simulink model "quad_model_control"  (R2025b)
settings: Solver=ode4  StartTime=0.0  StopTime=20  FixedStep=Ts/4  RelTol=1e-3
values from neighbouring files (symbols this model uses):
  axis_switch = [0 1 ... (first row only)    [quad_params.m]
  Cd = diag([0.10 0.10 0.15])    [quad_params.m]
  g = 9.81    [quad_params.m]
  Ivec = [Ixx; Iyy; Izz]    [quad_params.m]
  m = 1.20    (= 1.2)    [quad_params.m]
  MIX = [ kT     kT     kT     kT ... (first row only)    [quad_params.m]
  MIX_inv = inv(MIX)    [quad_params.m]
  ned_xy_kD = 1.92    [quad_params.m]
  ned_xy_kP = [1.44; 1.44]    [quad_params.m]
  ned_z_kD = 2.5    [quad_params.m]
  ned_z_kP = 2.7    [quad_params.m]
  om_dot_to_om = [0; 0; 0]    [quad_params.m]
  om_kP = [3;3;3]    [quad_params.m]
  p_ned_dot_to_p_ned = [0;0;0]    [quad_params.m]
  phi_dot_to_phi = [0;0;0]    [quad_params.m]
  pt1_w_cmd_to_w = zeros(4,1)    [quad_params.m]
  tau = 0.05    [quad_params.m]
  tau_kI = [0.125;0.125;0.324]    [quad_params.m]
  tau_kP = [0.10;0.10;0.216]    [quad_params.m]
  tau_sat_low = [-1.3;-1.3;-0.08]    [quad_params.m]
  tau_sat_up = [1.3;1.3;0.08]    [quad_params.m]
  Ts = 0.001    [quad_params.m]
  v_dot_to_v_b = [0;0;0]    [quad_params.m]
  w_max = 1200    [quad_params.m]
libraries: slpidlib x4
settings Model: Creator=chris  LastModifiedBy=chris
settings ModelReferenceCC: ModelReferenceMinAlgLoopOccurrences=on

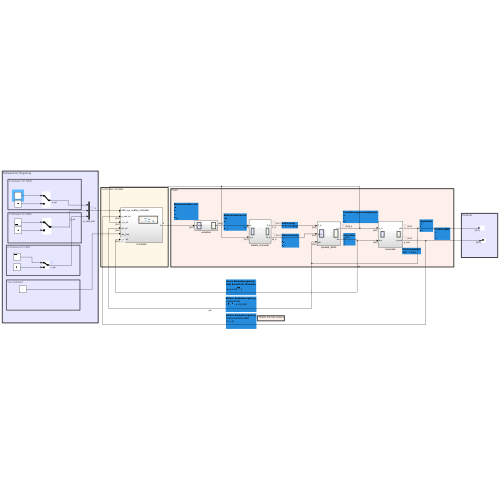
[thumbnail: Simulink's stored preview of the top-level diagram]
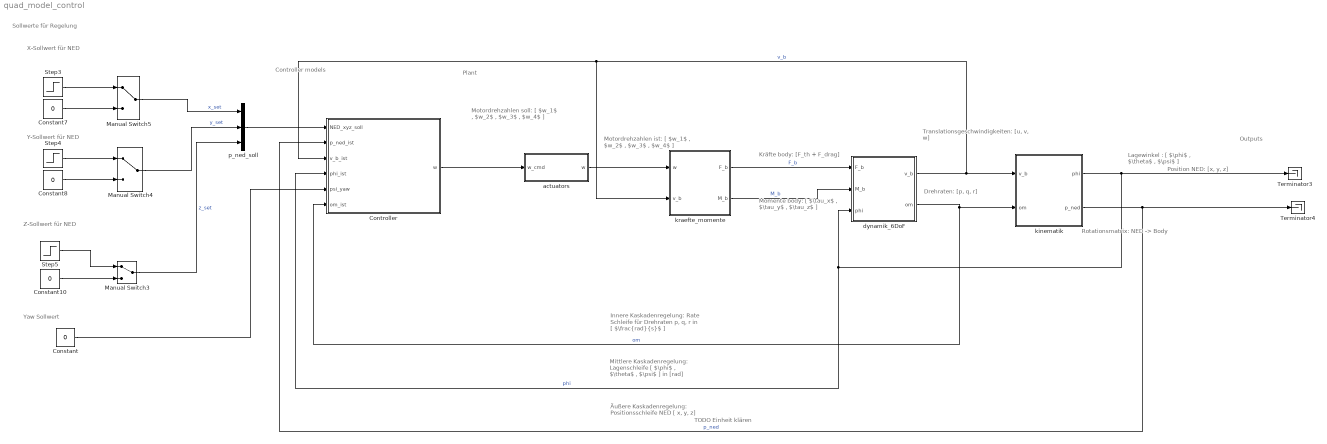
== system quad_model_control ==
  note: Controller models
  note: Plant
  note: Outputs
  note: Z-Sollwert für NED
  note: Sollwerte für Regelung
  note: Momente body:
      | [ $\tau_x$ ,
      | $\tau_y$ ,
      | $\tau_z$ ]
  note: Kräfte body:
      | [F_th + F_drag]
  note: Translationsgeschwindigkeiten:
      | [u,
      | v,
      | w]
  note: Drehraten:
      | [p,
      | q,
      | r]
  note: Lagewinkel :
      | [ $\phi$ ,
      | $\theta$ ,
      | $\psi$ ]
  note: Position NED:
      | [x,
      | y,
      | z]
  note: Rotationsmatrix:
      | NED -> Body
  note: Motordrehzahlen ist:
      | [ $w_1$ ,
      | $w_2$ ,
      | $w_3$ ,
      | $w_4$ ]
  note: Innere Kaskadenregelung:
      | Rate Schleife für Drehraten
      | p, q, r in [ $\frac{rad}{s}$ ]
  note: Mittlere Kaskadenregelung:
      | Lagenschleife
      | [ $\phi$ , $\theta$ , $\psi$ ] in [rad]
  note: Äußere Kaskadenregelung:
      | Positionsschleife NED
      | [ x, y, z]
  note: TODO Einheit klären
  note: X-Sollwert für NED
  note: Y-Sollwert für NED
  note: Motordrehzahlen soll:
      | [ $w_1$ ,
      | $w_2$ ,
      | $w_3$ ,
      | $w_4$ ]
  note: Yaw Sollwert
  Constant{,7..8,10} (4 alike) : Constant  Value=0
  Controller : Subsystem  Variant=on
  Manual Switch3 : ManualSwitch
  Manual Switch4 : ManualSwitch
  Manual Switch5 : ManualSwitch
  Step3 : Step  Time=2  After=2  SampleTime=0
  Step4 : Step  Time=2  After=2  SampleTime=0
  Step5 : Step  Time=2  After=-2  SampleTime=0
  Terminator3 : Terminator
  Terminator4 : Terminator
  actuators : Subsystem
  dynamik_6DoF : Subsystem
  kinematik : Subsystem
  kraefte_momente : Subsystem
  p_ned_soll : Mux  Inputs=3
  wires:
  dynamik_6DoF/2(om) -> Controller/6(om_ist), kinematik/2(om)  "om"
  kinematik/2(p_ned) -> Controller/2(p_ned_ist), Terminator4/1  "p_ned"
  kinematik/1(phi) -> dynamik_6DoF/3(phi), Controller/4(phi_ist), Terminator3/1  "phi"
  actuators/1(w) -> kraefte_momente/1(w)
  dynamik_6DoF/1(v_b) -> kinematik/1(v_b), Controller/3(v_b_ist), kraefte_momente/2(v_b)  "v_b"
  kraefte_momente/1(F_b) -> dynamik_6DoF/1(F_b)  "F_b"
  kraefte_momente/2(M_b) -> dynamik_6DoF/2(M_b)  "M_b"
  Constant8/1 -> Manual Switch4/2
  Step4/1 -> Manual Switch4/1
  Constant7/1 -> Manual Switch5/2
  Step3/1 -> Manual Switch5/1
  Manual Switch5/1 -> p_ned_soll/1  "x_set"
  Manual Switch4/1 -> p_ned_soll/2  "y_set"
  Step5/1 -> Manual Switch3/1
  Constant10/1 -> Manual Switch3/2
  Controller/1(w) -> actuators/1(w_cmd)
  p_ned_soll/1 -> Controller/1(NED_xyz_soll)
  Manual Switch3/1 -> p_ned_soll/3  "z_set"
  Constant/1 -> Controller/5(psi_yaw)

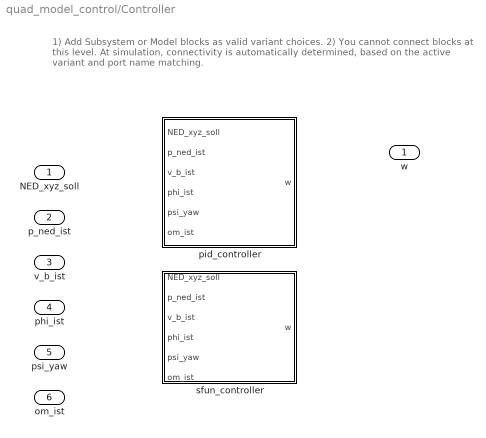
== system quad_model_control/Controller ==
  note: 1) Add Subsystem or Model blocks as valid variant choices.
      | 2) You cannot connect blocks at this level. At simulation, connectivity is automatically
      | determined, based on the active variant and port name matching.
  NED_xyz_soll : Inport
  p_ned_ist : Inport  Port=2
  v_b_ist : Inport  Port=3
  phi_ist : Inport  Port=4
  psi_yaw : Inport  Port=5
  om_ist : Inport  Port=6
  pid_controller : Subsystem  VariantControl=CTRL_IMPL ==1
  sfun_controller : Subsystem  VariantControl=CTRL_IMPL == 2
  w : Outport

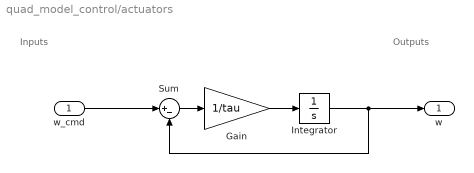
== system quad_model_control/actuators ==
  note: Inputs
  note: Outputs
  w_cmd : Inport  PortDimensions=[4 1]
  Gain : Gain  Gain=1/tau
  Integrator : Integrator  InitialCondition=pt1_w_cmd_to_w  LimitOutput=on  UpperSaturationLimit=w_max  LowerSaturationLimit=0  IgnoreLimit=on
  Sum : Sum  Inputs=|+-
  w : Outport  PortDimensions=[4 1]
  wires:
  Sum/1 -> Gain/1
  Gain/1 -> Integrator/1
  w_cmd/1 -> Sum/1
  Integrator/1 -> Sum/2, w/1

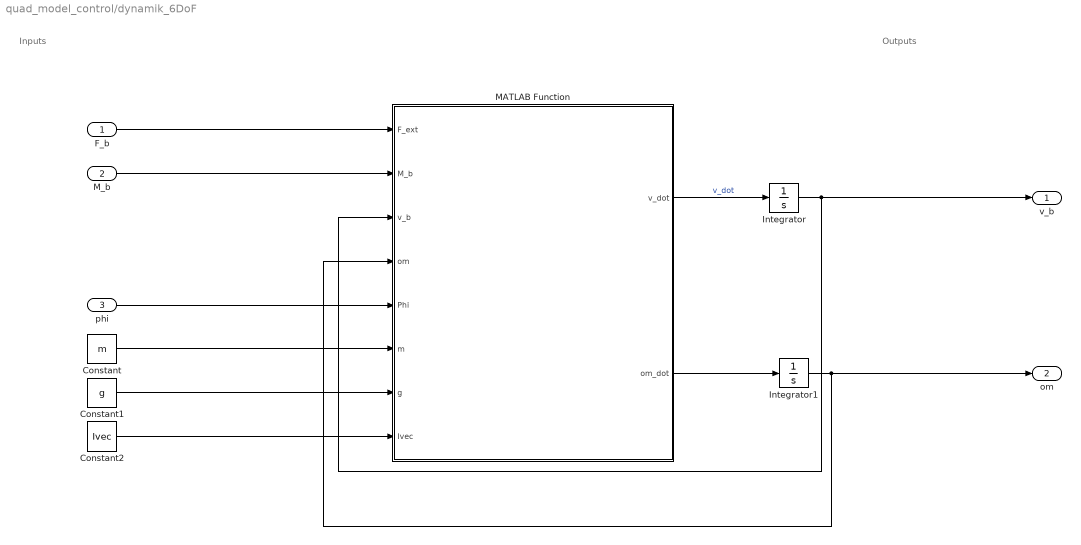
== system quad_model_control/dynamik_6DoF ==
  note: Inputs
  note: Outputs
  F_b : Inport  PortDimensions=[3 1]
  M_b : Inport  Port=2  PortDimensions=[3 1]
  phi : Inport  Port=3  PortDimensions=[3 1]
  Constant : Constant  Value=m
  Constant1 : Constant  Value=g
  Constant2 : Constant  Value=Ivec
  Integrator : Integrator  InitialCondition=v_dot_to_v_b
  Integrator1 : Integrator  InitialCondition=om_dot_to_om
  MATLAB Function : MATLAB Function  TreatAsAtomicUnit=on
  v_b : Outport  PortDimensions=[3 1]
  om : Outport  Port=2  PortDimensions=[3 1]
  wires:
  MATLAB Function/1(v_dot) -> Integrator/1  "v_dot"
  MATLAB Function/2(om_dot) -> Integrator1/1
  Constant1/1 -> MATLAB Function/7(g)
  F_b/1 -> MATLAB Function/1(F_ext)
  M_b/1 -> MATLAB Function/2(M_b)
  Constant/1 -> MATLAB Function/6(m)
  Integrator1/1 -> om/1, MATLAB Function/4(om)
  Constant2/1 -> MATLAB Function/8(Ivec)
  Integrator/1 -> v_b/1, MATLAB Function/3(v_b)
  phi/1 -> MATLAB Function/5(Phi)

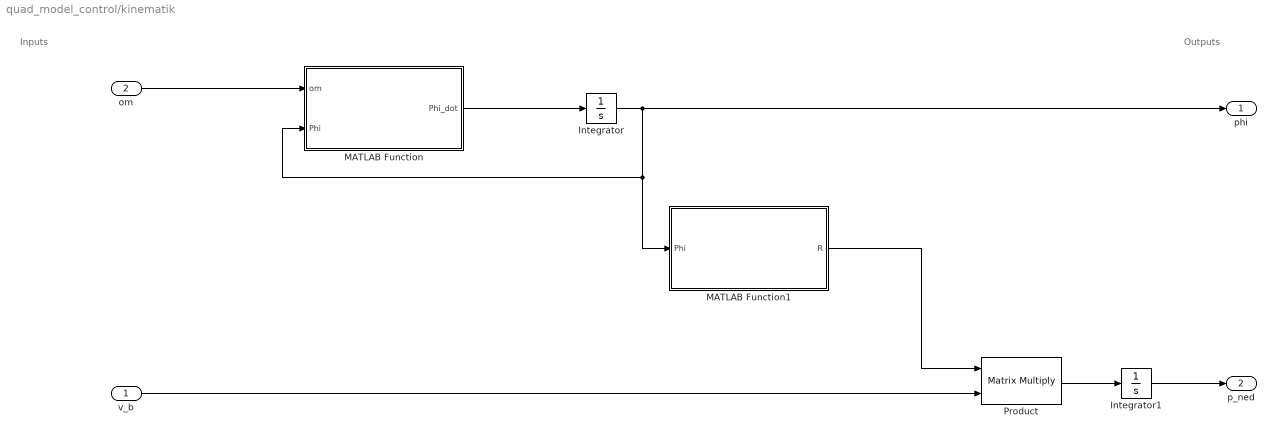
== system quad_model_control/kinematik ==
  note: Inputs
  note: Outputs
  v_b : Inport  PortDimensions=[3 1]
  om : Inport  Port=2  PortDimensions=[3 1]
  Integrator : Integrator  InitialCondition=phi_dot_to_phi
  Integrator1 : Integrator  InitialCondition=p_ned_dot_to_p_ned
  MATLAB Function : MATLAB Function  TreatAsAtomicUnit=on
  MATLAB Function1 : MATLAB Function  TreatAsAtomicUnit=on
  Product : Product  Multiplication=Matrix(*)
  phi : Outport  PortDimensions=[3 1]
  p_ned : Outport  Port=2
  wires:
  Integrator/1 -> phi/1, MATLAB Function1/1(Phi), MATLAB Function/2(Phi)
  Integrator1/1 -> p_ned/1
  v_b/1 -> Product/2
  MATLAB Function1/1(R) -> Product/1
  MATLAB Function/1(Phi_dot) -> Integrator/1
  om/1 -> MATLAB Function/1(om)
  Product/1 -> Integrator1/1

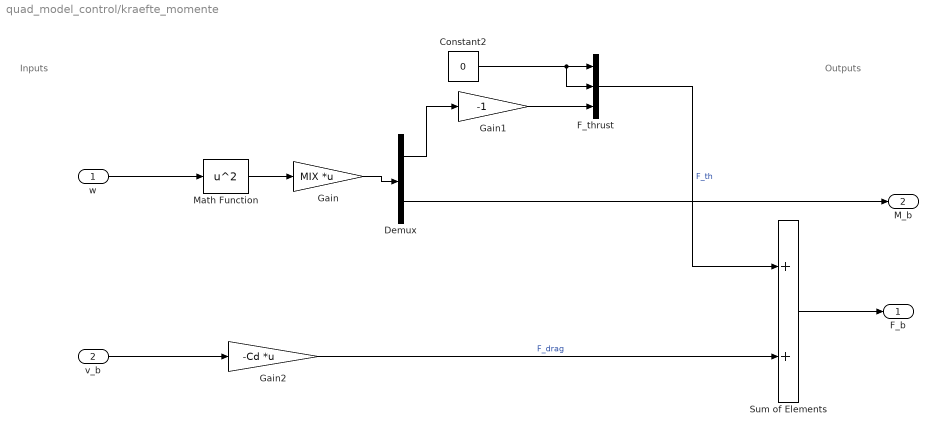
== system quad_model_control/kraefte_momente ==
  note: Inputs
  note: Outputs
  w : Inport  PortDimensions=[4 1]
  v_b : Inport  Port=2  PortDimensions=[3 1]
  Constant2 : Constant  Value=0
  Demux : Demux  Outputs=[1 3]
  F_thrust : Concatenate  NumInputs=3
  Gain : Gain  Gain=MIX  Multiplication=Matrix(K*u)
  Gain1 : Gain  Gain=-1
  Gain2 : Gain  Gain=-Cd  Multiplication=Matrix(K*u)
  Math Function : Math  Operator=square
  Sum of Elements : Sum
  F_b : Outport  PortDimensions=[3 1]
  M_b : Outport  Port=2  PortDimensions=[3 1]
  wires:
  v_b/1 -> Gain2/1
  Demux/2 -> M_b/1
  Constant2/1 -> F_thrust/2, F_thrust/1
  w/1 -> Math Function/1
  Gain2/1 -> Sum of Elements/2  "F_drag"
  Sum of Elements/1 -> F_b/1
  Math Function/1 -> Gain/1
  F_thrust/1 -> Sum of Elements/1  "F_th"
  Gain1/1 -> F_thrust/3
  Gain/1 -> Demux/1
  Demux/1 -> Gain1/1

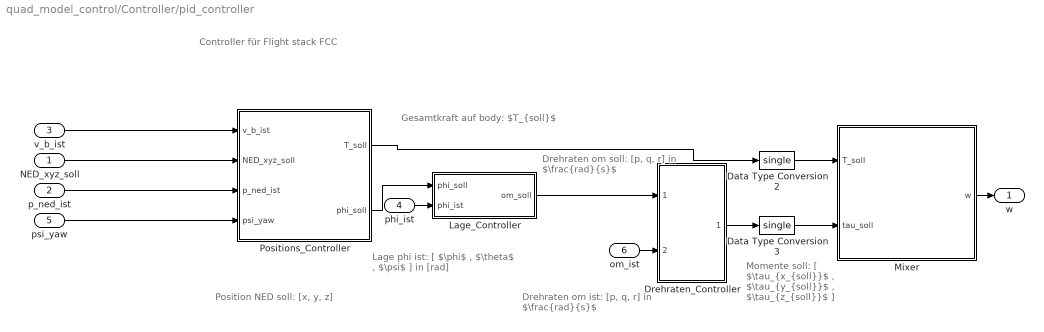
== system quad_model_control/Controller/pid_controller ==
  note: Controller für Flight stack FCC
  note: Drehraten om ist:
      | [p, q, r] in $\frac{rad}{s}$
  note: Lage phi ist:
      | [ $\phi$ , $\theta$ , $\psi$ ] in [rad]
  note: Momente soll:
      | [ $\tau_{x_{soll}}$ ,
      | $\tau_{y_{soll}}$ ,
      | $\tau_{z_{soll}}$ ]
  note: Gesamtkraft auf body:
      | $T_{soll}$
  note: Drehraten om soll:
      | [p, q, r] in $\frac{rad}{s}$
  note: Position NED soll:
      | [x, y, z]
  NED_xyz_soll : Inport
  p_ned_ist : Inport  Port=2
  v_b_ist : Inport  Port=3
  phi_ist : Inport  Port=4
  psi_yaw : Inport  Port=5
  om_ist : Inport  Port=6
  Data Type Conversion2 : DataTypeConversion  OutDataTypeStr=single  SaturateOnIntegerOverflow=off  RndMeth=Floor
  Data Type Conversion3 : DataTypeConversion  OutDataTypeStr=single  SaturateOnIntegerOverflow=off  RndMeth=Floor
  Drehraten_Controller : Subsystem
  Lage_Controller : Subsystem
  Mixer : Subsystem
  Positions_Controller : Subsystem
  w : Outport
  wires:
  psi_yaw/1 -> Positions_Controller/4(psi_yaw)
  Positions_Controller/2(phi_soll) -> Lage_Controller/1(phi_soll)
  Data Type Conversion2/1 -> Mixer/1(T_soll)
  Lage_Controller/1(om_soll) -> Drehraten_Controller/1(om_soll)
  Positions_Controller/1(T_soll) -> Data Type Conversion2/1
  Data Type Conversion3/1 -> Mixer/2(tau_soll)
  Mixer/1(w) -> w/1
  Drehraten_Controller/1(tau_soll) -> Data Type Conversion3/1
  phi_ist/1 -> Lage_Controller/2(phi_ist)
  v_b_ist/1 -> Positions_Controller/1(v_b_ist)
  p_ned_ist/1 -> Positions_Controller/3(p_ned_ist)
  om_ist/1 -> Drehraten_Controller/2(om_ist)
  NED_xyz_soll/1 -> Positions_Controller/2(NED_xyz_soll)

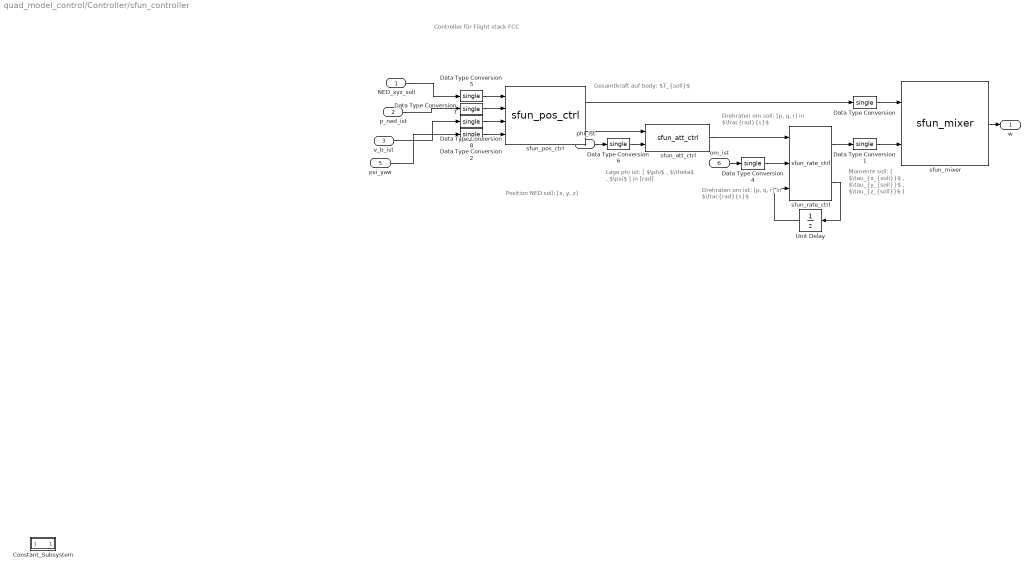
== system quad_model_control/Controller/sfun_controller ==
  note: Controller für Flight stack FCC
  note: Gesamtkraft auf body:
      | $T_{soll}$
  note: Drehraten om soll:
      | [p, q, r] in $\frac{rad}{s}$
  note: Drehraten om ist:
      | [p, q, r] in $\frac{rad}{s}$
  note: Lage phi ist:
      | [ $\phi$ , $\theta$ , $\psi$ ] in [rad]
  note: Position NED soll:
      | [x, y, z]
  note: Momente soll:
      | [ $\tau_{x_{soll}}$ ,
      | $\tau_{y_{soll}}$ ,
      | $\tau_{z_{soll}}$ ]
  NED_xyz_soll : Inport
  p_ned_ist : Inport  Port=2
  v_b_ist : Inport  Port=3
  phi_ist : Inport  Port=4
  psi_yaw : Inport  Port=5
  om_ist : Inport  Port=6
  Constant_Subsystem : Subsystem
  Data Type Conversion{,1..2,4..8} (8 alike) : DataTypeConversion  OutDataTypeStr=single  SaturateOnIntegerOverflow=off  RndMeth=Floor
  Unit Delay : UnitDelay  SampleTime=-1  HasFrameUpgradeWarning=on
  sfun_att_ctrl : S-Function  FunctionName=sfun_att_ctrl  SFunctionDeploymentMode=off  EnableBusSupport=off  mask(Legacy Function){SFunctionSpec=void att_ctrl_lct(single u1[3], single u2[3], single y1[3]), ShowSpec=on}
      mask prompts: ShowSpec "Display function specification"
      mask help:
      | This block allows you to call the legacy functions specified by the following Legacy Code Tool definition:
      | def.SFunctionName = 'sfun_att_ctrl';
      | def.OutputFcnSpec = 'void att_ctrl_lct(single u1[3], single u2[3], single y1[3])';
      | def.HeaderFiles = {'flight_ctrl_lct.h'};
      | def.SourceFiles = {'flight_ctrl.c', 'flight_ctrl_lct.c'};
      mask Help: <p>This block was generated automatically by the Legacy Code Tool. For detailed help on this tool, call<a href="matlab:legacy_code('help')"> legacy_code('help')</a>.</p>
      mask Callback ShowSpec:
      | if strcmp(get_param(gcbh, 'ShowSpec'), 'on')
      |   set_param(gcbh, 'MaskDisplay', sprintf('fprintf(''%s'');', get_param(gcbh, 'SFunctionSpec')));
      | else
      |   set_param(gcbh, 'MaskDisplay', sprintf('fprintf(''%s'');', get_param(gcbh, 'FunctionName')));
      | end
      mask Display: fprintf('void att_ctrl_lct(single u1[3], single u2[3], single y1[3])');
  sfun_mixer : S-Function  FunctionName=sfun_mixer  SFunctionDeploymentMode=off  EnableBusSupport=off  mask(Legacy Function){SFunctionSpec=void mixer_lct(single u1, single u2[3], single y1[4]), ShowSpec=on}
      mask prompts: ShowSpec "Display function specification"
      mask help:
      | This block allows you to call the legacy functions specified by the following Legacy Code Tool definition:
      | def.SFunctionName = 'sfun_mixer';
      | def.OutputFcnSpec = 'void mixer_lct(single u1, single u2[3], single y1[4])';
      | def.HeaderFiles = {'flight_ctrl_lct.h'};
      | def.SourceFiles = {'flight_ctrl.c', 'flight_ctrl_lct.c'};
      mask Help: <p>This block was generated automatically by the Legacy Code Tool. For detailed help on this tool, call<a href="matlab:legacy_code('help')"> legacy_code('help')</a>.</p>
      mask Callback ShowSpec:
      | if strcmp(get_param(gcbh, 'ShowSpec'), 'on')
      |   set_param(gcbh, 'MaskDisplay', sprintf('fprintf(''%s'');', get_param(gcbh, 'SFunctionSpec')));
      | else
      |   set_param(gcbh, 'MaskDisplay', sprintf('fprintf(''%s'');', get_param(gcbh, 'FunctionName')));
      | end
      mask Display: fprintf('void mixer_lct(single u1, single u2[3], single y1[4])');
  sfun_pos_ctrl : S-Function  FunctionName=sfun_pos_ctrl  SFunctionDeploymentMode=off  EnableBusSupport=off  mask(Legacy Function){SFunctionSpec=void pos_ctrl_lct(single u1[3], single u2[3], single u3[3], single u4, single y1[1], single y2[3]), ShowSpec=on}
      mask prompts: ShowSpec "Display function specification"
      mask help:
      | This block allows you to call the legacy functions specified by the following Legacy Code Tool definition:
      | def.SFunctionName = 'sfun_pos_ctrl';
      | def.OutputFcnSpec = 'void pos_ctrl_lct(single u1[3], single u2[3], single u3[3], single u4, single y1[1], single y2[3])';
      | def.HeaderFiles = {'flight_ctrl_lct.h'};
      | def.SourceFiles = {'flight_ctrl.c', 'flight_ctrl_lct.c'};
      mask Help: <p>This block was generated automatically by the Legacy Code Tool. For detailed help on this tool, call<a href="matlab:legacy_code('help')"> legacy_code('help')</a>.</p>
      mask Callback ShowSpec:
      | if strcmp(get_param(gcbh, 'ShowSpec'), 'on')
      |   set_param(gcbh, 'MaskDisplay', sprintf('fprintf(''%s'');', get_param(gcbh, 'SFunctionSpec')));
      | else
      |   set_param(gcbh, 'MaskDisplay', sprintf('fprintf(''%s'');', get_param(gcbh, 'FunctionName')));
      | end
      mask Display: fprintf('void pos_ctrl_lct(single u1[3], single u2[3], single u3[3], single u4, single y1[1], single y2[3])');
  sfun_rate_ctrl : S-Function  FunctionName=sfun_rate_ctrl  SFunctionDeploymentMode=off  EnableBusSupport=off  mask(Legacy Function){SFunctionSpec=void rate_ctrl_lct(single u1[3], single u2[3], single u3[3], single y1[3], single y2[3]), ShowSpec=on}
      mask prompts: ShowSpec "Display function specification"
      mask help:
      | This block allows you to call the legacy functions specified by the following Legacy Code Tool definition:
      | def.SFunctionName = 'sfun_rate_ctrl';
      | def.OutputFcnSpec = 'void rate_ctrl_lct(single u1[3], single u2[3], single u3[3], single y1[3], single y2[3])';
      | def.HeaderFiles = {'flight_ctrl_lct.h'};
      | def.SourceFiles = {'flight_ctrl.c', 'flight_ctrl_lct.c'};
      mask Help: <p>This block was generated automatically by the Legacy Code Tool. For detailed help on this tool, call<a href="matlab:legacy_code('help')"> legacy_code('help')</a>.</p>
      mask Callback ShowSpec:
      | if strcmp(get_param(gcbh, 'ShowSpec'), 'on')
      |   set_param(gcbh, 'MaskDisplay', sprintf('fprintf(''%s'');', get_param(gcbh, 'SFunctionSpec')));
      | else
      |   set_param(gcbh, 'MaskDisplay', sprintf('fprintf(''%s'');', get_param(gcbh, 'FunctionName')));
      | end
      mask Display: fprintf('void rate_ctrl_lct(single u1[3], single u2[3], single u3[3], single y1[3], single y2[3])');
  w : Outport
  wires:
  Data Type Conversion7/1 -> sfun_pos_ctrl/2
  sfun_att_ctrl/1 -> sfun_rate_ctrl/1
  Data Type Conversion5/1 -> sfun_pos_ctrl/1
  sfun_rate_ctrl/1 -> Data Type Conversion1/1
  Data Type Conversion/1 -> sfun_mixer/1
  NED_xyz_soll/1 -> Data Type Conversion5/1
  Data Type Conversion4/1 -> sfun_rate_ctrl/2
  Data Type Conversion6/1 -> sfun_att_ctrl/2
  Data Type Conversion1/1 -> sfun_mixer/2
  om_ist/1 -> Data Type Conversion4/1
  sfun_pos_ctrl/1 -> Data Type Conversion/1
  Data Type Conversion8/1 -> sfun_pos_ctrl/3
  Unit Delay/1 -> sfun_rate_ctrl/3
  v_b_ist/1 -> Data Type Conversion8/1
  sfun_rate_ctrl/2 -> Unit Delay/1
  sfun_pos_ctrl/2 -> sfun_att_ctrl/1
  sfun_mixer/1 -> w/1
  phi_ist/1 -> Data Type Conversion6/1
  p_ned_ist/1 -> Data Type Conversion7/1
  psi_yaw/1 -> Data Type Conversion2/1
  Data Type Conversion2/1 -> sfun_pos_ctrl/4

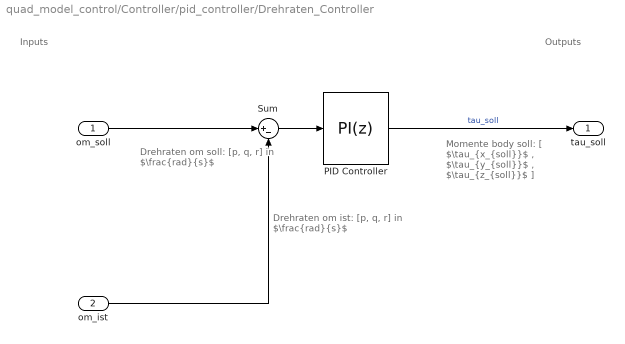
== system quad_model_control/Controller/pid_controller/Drehraten_Controller ==
  note: Inputs
  note: Momente body
      | soll:
      | [ $\tau_{x_{soll}}$ ,
      | $\tau_{y_{soll}}$ ,
      | $\tau_{z_{soll}}$ ]
  note: Drehraten om ist:
      | [p, q, r] in $\frac{rad}{s}$
  note: Drehraten om soll:
      | [p, q, r] in $\frac{rad}{s}$
  note: Outputs
  om_soll : Inport
  om_ist : Inport  Port=2
  PID Controller : slpidlib/PID Controller  Controller=PI  Form=Parallel  TimeDomain=Discrete-time  UseExternalTs=off  SampleTime=Ts  IntegratorMethod=Backward Euler  FilterMethod=Forward Euler  ControllerParametersSource=internal  P=tau_kP  I=tau_kI  UseKiTs=off  D=0  UseExternalDerivativeSource=off  N=100  UseFilter=on  TunerSelectOption=Transfer Function Based (PID Tuner App)  InitialConditionSource=internal  InitialConditionForIntegrator=0  InitialConditionForFilter=0  DifferentiatorICPrevScaledInput=0  ExternalReset=none  TrackingMode=off  Kt=1  LimitOutput=on  SatLimitsSource=internal  UpperSaturationLimit=tau_sat_up  LowerSaturationLimit=tau_sat_low  LinearizeAsGain=on  AntiWindupMode=clamping  Kb=1  LimitIntegrator=off  UpperIntegratorSaturationLimit=inf  LowerIntegratorSaturationLimit=-inf  POutMin=[]  POutMax=[]  IOutMin=[]  IOutMax=[]  DOutMin=[]  DOutMax=[]  NOutMin=[]  NOutMax=[]  SumOutMin=[]  SumOutMax=[]  SaturationOutMin=[]  SaturationOutMax=[]  PParamMin=[]  PParamMax=[]  IParamMin=[]  IParamMax=[]  DParamMin=[]  DParamMax=[]  NParamMin=[]  NParamMax=[]  KbParamMin=[]  KbParamMax=[]  KtParamMin=[]  KtParamMax=[]  KbOutMin=[]  KbOutMax=[]  KtOutMin=[]  KtOutMax=[]  IntegratorOutMin=[]  IntegratorOutMax=[]  FilterOutMin=[]  FilterOutMax=[]  SumI1OutMin=[]  SumI1OutMax=[]  SumI2OutMin=[]  SumI2OutMax=[]  SumI3OutMin=[]  SumI3OutMax=[]  SumI4OutMin=[]  SumI4OutMax=[]  SumDOutMin=[]  SumDOutMax=[]  DifferentiatorOutMin=[]  DifferentiatorOutMax=[]  FilterDiffOutCoefMin=[]  FilterDiffOutCoefMax=[]  ReciprocalOutMin=[]  ReciprocalOutMax=[]  SumDenOutMin=[]  SumDenOutMax=[]  SumNumOutMin=[]  SumNumOutMax=[]  DivideOutMin=[]  DivideOutMax=[]  UdiffTsProdOutMin=[]  UdiffTsProdOutMax=[]  NTsProdOutMin=[]  NTsProdOutMax=[]  UintegralTsProdOutMin=[]  UintegralTsProdOutMax=[]  UngainTsProdOutMin=[]  UngainTsProdOutMax=[]  ClampingZeroOutDataTypeStr=Inherit: Inherit via back propagation  ClampingZeroOutMin=[]  ClampingZeroOutMax=[]  FilterDenConstantOutDataTypeStr=Inherit: Inherit via back propagation  FilterDenConstantOutMin=[]  FilterDenConstantOutMax=[]  PCopyOutDataTypeStr=Inherit: Inherit via back propagation  PCopyOutMin=[]  PCopyOutMax=[]  NCopyOutDataTypeStr=Inherit: Inherit via back propagation  NCopyOutMin=[]  NCopyOutMax=[]  IntegratorContinuousStateAttributes=''  IntegratorStateMustResolveToSignalObject=off  IntegratorRTWStateStorageClass=Auto  FilterContinuousStateAttributes=''  FilterStateMustResolveToSignalObject=off  FilterRTWStateStorageClass=Auto  ParallelPVariant=InternalParameters  IdealPVariant=Disabled  IVariant=InternalParameters  DVariant=Disabled  IntegratorVariant=Discrete  SatVariant=Enabled  AWVariant=DiscClampingParallel  PCopyVariant=Disabled  TRVariant=Disabled  FdbkBlocksVariant=Feedback  IdealPFdbkVariant=Passthrough  SatFdbkVariant=Passthrough  DerivativeFilterVariant=Disabled  NVariant=Disabled  NCopyVariant=Disabled_SignalSpec  FilterICVariant=Disabled  IntegratorICVariant=InternalICs  ExternalResetVariant=Disabled  TRSumVariant=Passthrough  SumFdbkVariant=Enabled  SumVariant=Sum_PI  TsampFilterVariant=InternalTs  TsampNgainVariant=Passthrough  TsampIntegralVariant=Disabled_SignalSpec  ExternalSaturationOutDataTypeStr=Inherit: Same as second input  DerivativeSourceVariant=Disabled  PreIntVariant=InternalPreInt
  Sum : Sum  Inputs=|+-
  tau_soll : Outport  PortDimensions=[3 1]
  wires:
  om_soll/1 -> Sum/1
  Sum/1 -> PID Controller/1
  PID Controller/1 -> tau_soll/1  "tau_soll"
  om_ist/1 -> Sum/2

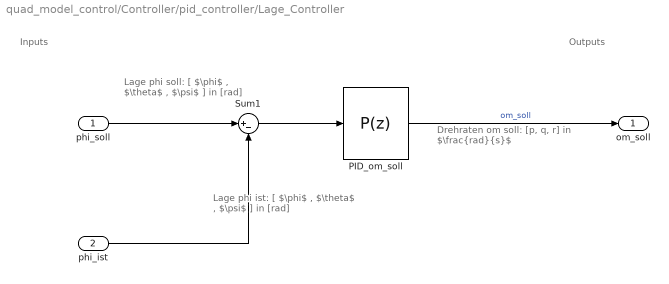
== system quad_model_control/Controller/pid_controller/Lage_Controller ==
  note: Inputs
  note: Drehraten om soll:
      | [p, q, r] in $\frac{rad}{s}$
  note: Lage phi soll:
      | [ $\phi$ , $\theta$ , $\psi$ ] in [rad]
  note: Lage phi ist:
      | [ $\phi$ , $\theta$ , $\psi$ ] in [rad]
  note: Outputs
  phi_soll : Inport
  phi_ist : Inport  Port=2
  PID_om_soll : slpidlib/PID Controller  Controller=P  Form=Parallel  TimeDomain=Discrete-time  UseExternalTs=off  SampleTime=Ts  IntegratorMethod=Forward Euler  FilterMethod=Forward Euler  ControllerParametersSource=internal  P=om_kP  I=0  UseKiTs=off  D=0  UseExternalDerivativeSource=off  N=100  UseFilter=on  TunerSelectOption=Transfer Function Based (PID Tuner App)  InitialConditionSource=internal  InitialConditionForIntegrator=0  InitialConditionForFilter=0  DifferentiatorICPrevScaledInput=0  ExternalReset=none  TrackingMode=off  Kt=1  LimitOutput=on  SatLimitsSource=internal  UpperSaturationLimit=inf  LowerSaturationLimit=-inf  LinearizeAsGain=on  AntiWindupMode=clamping  Kb=1  LimitIntegrator=off  UpperIntegratorSaturationLimit=inf  LowerIntegratorSaturationLimit=-inf  POutMin=[]  POutMax=[]  IOutMin=[]  IOutMax=[]  DOutMin=[]  DOutMax=[]  NOutMin=[]  NOutMax=[]  SumOutMin=[]  SumOutMax=[]  SaturationOutMin=[]  SaturationOutMax=[]  PParamMin=[]  PParamMax=[]  IParamMin=[]  IParamMax=[]  DParamMin=[]  DParamMax=[]  NParamMin=[]  NParamMax=[]  KbParamMin=[]  KbParamMax=[]  KtParamMin=[]  KtParamMax=[]  KbOutMin=[]  KbOutMax=[]  KtOutMin=[]  KtOutMax=[]  IntegratorOutMin=[]  IntegratorOutMax=[]  FilterOutMin=[]  FilterOutMax=[]  SumI1OutMin=[]  SumI1OutMax=[]  SumI2OutMin=[]  SumI2OutMax=[]  SumI3OutMin=[]  SumI3OutMax=[]  SumI4OutMin=[]  SumI4OutMax=[]  SumDOutMin=[]  SumDOutMax=[]  DifferentiatorOutMin=[]  DifferentiatorOutMax=[]  FilterDiffOutCoefMin=[]  FilterDiffOutCoefMax=[]  ReciprocalOutMin=[]  ReciprocalOutMax=[]  SumDenOutMin=[]  SumDenOutMax=[]  SumNumOutMin=[]  SumNumOutMax=[]  DivideOutMin=[]  DivideOutMax=[]  UdiffTsProdOutMin=[]  UdiffTsProdOutMax=[]  NTsProdOutMin=[]  NTsProdOutMax=[]  UintegralTsProdOutMin=[]  UintegralTsProdOutMax=[]  UngainTsProdOutMin=[]  UngainTsProdOutMax=[]  ClampingZeroOutDataTypeStr=Inherit: Inherit via back propagation  ClampingZeroOutMin=[]  ClampingZeroOutMax=[]  FilterDenConstantOutDataTypeStr=Inherit: Inherit via back propagation  FilterDenConstantOutMin=[]  FilterDenConstantOutMax=[]  PCopyOutDataTypeStr=Inherit: Inherit via back propagation  PCopyOutMin=[]  PCopyOutMax=[]  NCopyOutDataTypeStr=Inherit: Inherit via back propagation  NCopyOutMin=[]  NCopyOutMax=[]  IntegratorContinuousStateAttributes=''  IntegratorStateMustResolveToSignalObject=off  IntegratorRTWStateStorageClass=Auto  FilterContinuousStateAttributes=''  FilterStateMustResolveToSignalObject=off  FilterRTWStateStorageClass=Auto  ParallelPVariant=InternalParameters  IdealPVariant=Disabled  IVariant=Disabled  DVariant=Disabled  IntegratorVariant=Disabled  SatVariant=Enabled  AWVariant=Disabled  PCopyVariant=Disabled  TRVariant=Disabled  FdbkBlocksVariant=Forward  IdealPFdbkVariant=Disabled  SatFdbkVariant=Disabled  DerivativeFilterVariant=Disabled  NVariant=Disabled  NCopyVariant=Disabled_SignalSpec  FilterICVariant=Disabled  IntegratorICVariant=Disabled  ExternalResetVariant=Disabled  TRSumVariant=Passthrough  SumFdbkVariant=Disabled  SumVariant=Passthrough_P  TsampFilterVariant=InternalTs  TsampNgainVariant=Passthrough  TsampIntegralVariant=Disabled_SignalSpec  ExternalSaturationOutDataTypeStr=Inherit: Same as second input  DerivativeSourceVariant=Disabled  PreIntVariant=InternalPreInt
  Sum1 : Sum  Inputs=|+-
  om_soll : Outport
  wires:
  PID_om_soll/1 -> om_soll/1  "om_soll"
  Sum1/1 -> PID_om_soll/1
  phi_ist/1 -> Sum1/2
  phi_soll/1 -> Sum1/1

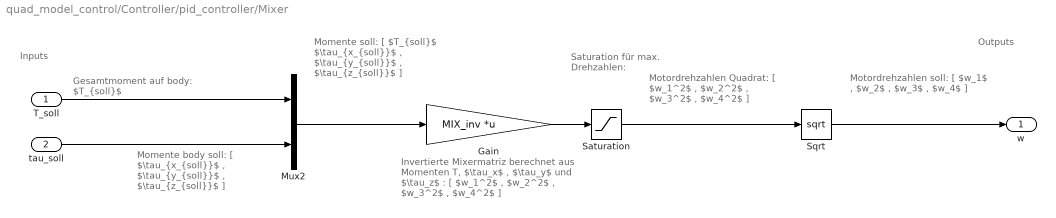
== system quad_model_control/Controller/pid_controller/Mixer ==
  note: Inputs
  note: Motordrehzahlen soll:
      | [ $w_1$ ,
      | $w_2$ ,
      | $w_3$ ,
      | $w_4$ ]
  note: Motordrehzahlen Quadrat:
      | [ $w_1^2$ ,
      | $w_2^2$ ,
      | $w_3^2$ ,
      | $w_4^2$ ]
  note: Invertierte Mixermatriz berechnet aus
      | Momenten T, $\tau_x$ , $\tau_y$ und $\tau_z$ :
      | [ $w_1^2$ ,
      | $w_2^2$ ,
      | $w_3^2$ ,
      | $w_4^2$ ]
  note: Saturation
      | für max.
      | Drehzahlen:
  note: Outputs
  note: Momente soll:
      | [ $T_{soll}$
      | $\tau_{x_{soll}}$ ,
      | $\tau_{y_{soll}}$ ,
      | $\tau_{z_{soll}}$ ]
  note: Gesamtmoment auf body:
      | $T_{soll}$
  note: Momente body
      | soll:
      | [ $\tau_{x_{soll}}$ ,
      | $\tau_{y_{soll}}$ ,
      | $\tau_{z_{soll}}$ ]
  T_soll : Inport
  tau_soll : Inport  Port=2  PortDimensions=[3 1]
  Gain : Gain  Gain=MIX_inv  Multiplication=Matrix(K*u)
  Mux2 : Mux  Inputs=2
  Saturation : Saturate  UpperLimit=w_max^2  LowerLimit=0
  Sqrt : Sqrt
  w : Outport
  wires:
  Mux2/1 -> Gain/1
  Gain/1 -> Saturation/1
  Sqrt/1 -> w/1
  Saturation/1 -> Sqrt/1
  T_soll/1 -> Mux2/1
  tau_soll/1 -> Mux2/2

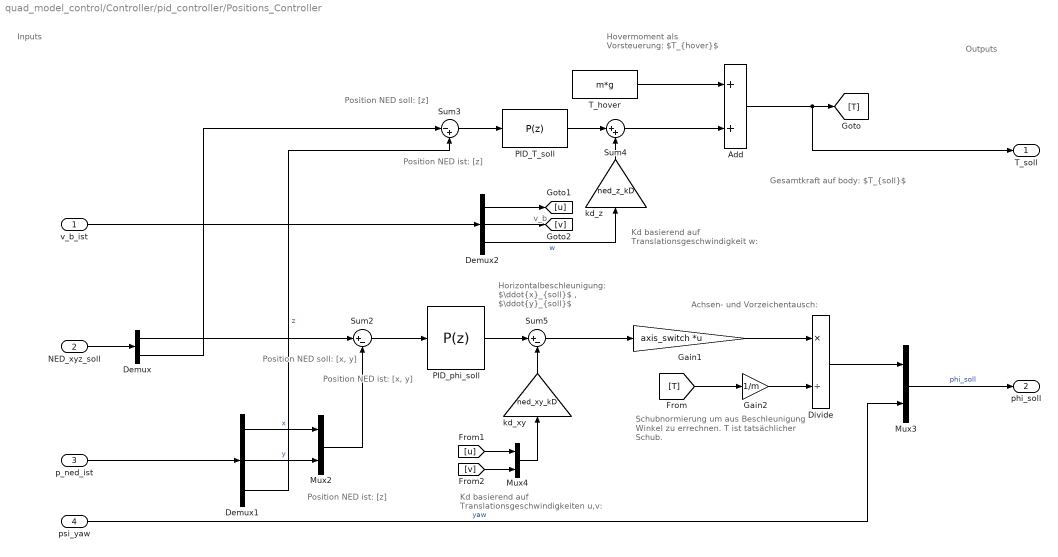
== system quad_model_control/Controller/pid_controller/Positions_Controller ==
  note: Inputs
  note: v_b
  note: Position NED soll:
      | [x, y]
  note: Position NED ist:
      | [x, y]
  note: Position NED ist:
      | [z]
  note: Position NED ist:
      | [z]
  note: Position NED soll:
      | [z]
  note: Gesamtkraft auf body:
      | $T_{soll}$
  note: Hovermoment als Vorsteuerung:
      | $T_{hover}$
  note: Kd basierend auf Translationsgeschwindigkeit w:
  note: Horizontalbeschleunigung:
      | $\ddot{x}_{soll}$ , $\ddot{y}_{soll}$
  note: Achsen- und Vorzeichentausch:
  note: Schubnormierung um aus Beschleunigung Winkel zu errechnen. T ist tatsächlicher Schub.
  note: Kd basierend auf Translationsgeschwindigkeiten u,v:
  note: Outputs
  v_b_ist : Inport
  NED_xyz_soll : Inport  Port=2
  p_ned_ist : Inport  Port=3
  psi_yaw : Inport  Port=4
  Add : Sum
  Demux : Demux  Outputs=2
  Demux1 : Demux  Outputs=3
  Demux2 : Demux  Outputs=3
  Divide : Product  Inputs=*/
  Gain1 : Gain  Gain=axis_switch  Multiplication=Matrix(K*u)
  Gain2 : Gain  Gain=1/m
  Mux2 : Mux  Inputs=2
  Mux3 : Mux  Inputs=2
  Mux4 : Mux  Inputs=2
  PID_T_soll : slpidlib/PID Controller  Controller=P  Form=Parallel  TimeDomain=Discrete-time  UseExternalTs=off  SampleTime=Ts  IntegratorMethod=Forward Euler  FilterMethod=Forward Euler  ControllerParametersSource=internal  P=ned_z_kP  I=0  UseKiTs=off  D=0  UseExternalDerivativeSource=off  N=100  UseFilter=on  TunerSelectOption=Transfer Function Based (PID Tuner App)  InitialConditionSource=internal  InitialConditionForIntegrator=0  InitialConditionForFilter=0  DifferentiatorICPrevScaledInput=0  ExternalReset=none  TrackingMode=off  Kt=1  LimitOutput=on  SatLimitsSource=internal  UpperSaturationLimit=inf  LowerSaturationLimit=-inf  LinearizeAsGain=on  AntiWindupMode=clamping  Kb=1  LimitIntegrator=off  UpperIntegratorSaturationLimit=inf  LowerIntegratorSaturationLimit=-inf  POutMin=[]  POutMax=[]  IOutMin=[]  IOutMax=[]  DOutMin=[]  DOutMax=[]  NOutMin=[]  NOutMax=[]  SumOutMin=[]  SumOutMax=[]  SaturationOutMin=[]  SaturationOutMax=[]  PParamMin=[]  PParamMax=[]  IParamMin=[]  IParamMax=[]  DParamMin=[]  DParamMax=[]  NParamMin=[]  NParamMax=[]  KbParamMin=[]  KbParamMax=[]  KtParamMin=[]  KtParamMax=[]  KbOutMin=[]  KbOutMax=[]  KtOutMin=[]  KtOutMax=[]  IntegratorOutMin=[]  IntegratorOutMax=[]  FilterOutMin=[]  FilterOutMax=[]  SumI1OutMin=[]  SumI1OutMax=[]  SumI2OutMin=[]  SumI2OutMax=[]  SumI3OutMin=[]  SumI3OutMax=[]  SumI4OutMin=[]  SumI4OutMax=[]  SumDOutMin=[]  SumDOutMax=[]  DifferentiatorOutMin=[]  DifferentiatorOutMax=[]  FilterDiffOutCoefMin=[]  FilterDiffOutCoefMax=[]  ReciprocalOutMin=[]  ReciprocalOutMax=[]  SumDenOutMin=[]  SumDenOutMax=[]  SumNumOutMin=[]  SumNumOutMax=[]  DivideOutMin=[]  DivideOutMax=[]  UdiffTsProdOutMin=[]  UdiffTsProdOutMax=[]  NTsProdOutMin=[]  NTsProdOutMax=[]  UintegralTsProdOutMin=[]  UintegralTsProdOutMax=[]  UngainTsProdOutMin=[]  UngainTsProdOutMax=[]  ClampingZeroOutDataTypeStr=Inherit: Inherit via back propagation  ClampingZeroOutMin=[]  ClampingZeroOutMax=[]  FilterDenConstantOutDataTypeStr=Inherit: Inherit via back propagation  FilterDenConstantOutMin=[]  FilterDenConstantOutMax=[]  PCopyOutDataTypeStr=Inherit: Inherit via back propagation  PCopyOutMin=[]  PCopyOutMax=[]  NCopyOutDataTypeStr=Inherit: Inherit via back propagation  NCopyOutMin=[]  NCopyOutMax=[]  IntegratorContinuousStateAttributes=''  IntegratorStateMustResolveToSignalObject=off  IntegratorRTWStateStorageClass=Auto  FilterContinuousStateAttributes=''  FilterStateMustResolveToSignalObject=off  FilterRTWStateStorageClass=Auto  ParallelPVariant=InternalParameters  IdealPVariant=Disabled  IVariant=Disabled  DVariant=Disabled  IntegratorVariant=Disabled  SatVariant=Enabled  AWVariant=Disabled  PCopyVariant=Disabled  TRVariant=Disabled  FdbkBlocksVariant=Forward  IdealPFdbkVariant=Disabled  SatFdbkVariant=Disabled  DerivativeFilterVariant=Disabled  NVariant=Disabled  NCopyVariant=Disabled_SignalSpec  FilterICVariant=Disabled  IntegratorICVariant=Disabled  ExternalResetVariant=Disabled  TRSumVariant=Passthrough  SumFdbkVariant=Disabled  SumVariant=Passthrough_P  TsampFilterVariant=InternalTs  TsampNgainVariant=Passthrough  TsampIntegralVariant=Disabled_SignalSpec  ExternalSaturationOutDataTypeStr=Inherit: Same as second input  DerivativeSourceVariant=Disabled  PreIntVariant=InternalPreInt
  PID_phi_soll : slpidlib/PID Controller  Controller=P  Form=Parallel  TimeDomain=Discrete-time  UseExternalTs=off  SampleTime=Ts  IntegratorMethod=Forward Euler  FilterMethod=Forward Euler  ControllerParametersSource=internal  P=ned_xy_kP  I=0  UseKiTs=off  D=[1.37, 1.37]  UseExternalDerivativeSource=off  N=100  UseFilter=on  TunerSelectOption=Transfer Function Based (PID Tuner App)  InitialConditionSource=internal  InitialConditionForIntegrator=0  InitialConditionForFilter=0  DifferentiatorICPrevScaledInput=0  ExternalReset=none  TrackingMode=off  Kt=1  LimitOutput=on  SatLimitsSource=internal  UpperSaturationLimit=inf  LowerSaturationLimit=-inf  LinearizeAsGain=on  AntiWindupMode=clamping  Kb=1  LimitIntegrator=off  UpperIntegratorSaturationLimit=inf  LowerIntegratorSaturationLimit=-inf  POutMin=[]  POutMax=[]  IOutMin=[]  IOutMax=[]  DOutMin=[]  DOutMax=[]  NOutMin=[]  NOutMax=[]  SumOutMin=[]  SumOutMax=[]  SaturationOutMin=[]  SaturationOutMax=[]  PParamMin=[]  PParamMax=[]  IParamMin=[]  IParamMax=[]  DParamMin=[]  DParamMax=[]  NParamMin=[]  NParamMax=[]  KbParamMin=[]  KbParamMax=[]  KtParamMin=[]  KtParamMax=[]  KbOutMin=[]  KbOutMax=[]  KtOutMin=[]  KtOutMax=[]  IntegratorOutMin=[]  IntegratorOutMax=[]  FilterOutMin=[]  FilterOutMax=[]  SumI1OutMin=[]  SumI1OutMax=[]  SumI2OutMin=[]  SumI2OutMax=[]  SumI3OutMin=[]  SumI3OutMax=[]  SumI4OutMin=[]  SumI4OutMax=[]  SumDOutMin=[]  SumDOutMax=[]  DifferentiatorOutMin=[]  DifferentiatorOutMax=[]  FilterDiffOutCoefMin=[]  FilterDiffOutCoefMax=[]  ReciprocalOutMin=[]  ReciprocalOutMax=[]  SumDenOutMin=[]  SumDenOutMax=[]  SumNumOutMin=[]  SumNumOutMax=[]  DivideOutMin=[]  DivideOutMax=[]  UdiffTsProdOutMin=[]  UdiffTsProdOutMax=[]  NTsProdOutMin=[]  NTsProdOutMax=[]  UintegralTsProdOutMin=[]  UintegralTsProdOutMax=[]  UngainTsProdOutMin=[]  UngainTsProdOutMax=[]  ClampingZeroOutDataTypeStr=Inherit: Inherit via back propagation  ClampingZeroOutMin=[]  ClampingZeroOutMax=[]  FilterDenConstantOutDataTypeStr=Inherit: Inherit via back propagation  FilterDenConstantOutMin=[]  FilterDenConstantOutMax=[]  PCopyOutDataTypeStr=Inherit: Inherit via back propagation  PCopyOutMin=[]  PCopyOutMax=[]  NCopyOutDataTypeStr=Inherit: Inherit via back propagation  NCopyOutMin=[]  NCopyOutMax=[]  IntegratorContinuousStateAttributes=''  IntegratorStateMustResolveToSignalObject=off  IntegratorRTWStateStorageClass=Auto  FilterContinuousStateAttributes=''  FilterStateMustResolveToSignalObject=off  FilterRTWStateStorageClass=Auto  ParallelPVariant=InternalParameters  IdealPVariant=Disabled  IVariant=Disabled  DVariant=Disabled  IntegratorVariant=Disabled  SatVariant=Enabled  AWVariant=Disabled  PCopyVariant=Disabled  TRVariant=Disabled  FdbkBlocksVariant=Forward  IdealPFdbkVariant=Disabled  SatFdbkVariant=Disabled  DerivativeFilterVariant=Disabled  NVariant=Disabled  NCopyVariant=Disabled_SignalSpec  FilterICVariant=Disabled  IntegratorICVariant=Disabled  ExternalResetVariant=Disabled  TRSumVariant=Passthrough  SumFdbkVariant=Disabled  SumVariant=Passthrough_P  TsampFilterVariant=InternalTs  TsampNgainVariant=Passthrough  TsampIntegralVariant=Disabled_SignalSpec  ExternalSaturationOutDataTypeStr=Inherit: Same as second input  DerivativeSourceVariant=Disabled  PreIntVariant=InternalPreInt
  Sum2 : Sum  Inputs=|+-
  Sum3 : Sum  Inputs=|-+
  Sum4 : Sum  Inputs=|++
  Sum5 : Sum  Inputs=|+-
  T_hover : Constant  Value=m*g
  kd_xy : Gain  Gain=ned_xy_kD
  kd_z : Gain  Gain=ned_z_kD
  T_soll : Outport
  phi_soll : Outport  Port=2
  wires:
  Mux2/1 -> Sum2/2
  Add/1 -> T_soll/1, [T]
  Divide/1 -> Mux3/1
  Mux4/1 -> kd_xy/1
  p_ned_ist/1 -> Demux1/1
  Sum3/1 -> PID_T_soll/1
  PID_T_soll/1 -> Sum4/1
  Demux2/3 -> kd_z/1  "w"
  Sum2/1 -> PID_phi_soll/1
  Gain2/1 -> Divide/2
  Sum4/1 -> Add/2
  Demux1/1 -> Mux2/1  "x"
  Demux1/2 -> Mux2/2  "y"
  kd_z/1 -> Sum4/2
  [T] -> Gain2/1
  T_hover/1 -> Add/1
  Demux1/3 -> Sum3/2  "z"
  Gain1/1 -> Divide/1
  Sum5/1 -> Gain1/1
  psi_yaw/1 -> Mux3/2  "yaw"
  Demux2/1 -> [u]
  kd_xy/1 -> Sum5/2
  Demux2/2 -> [v]
  [u] -> Mux4/1
  [v] -> Mux4/2
  PID_phi_soll/1 -> Sum5/1
  Mux3/1 -> phi_soll/1  "phi_soll"
  v_b_ist/1 -> Demux2/1
  NED_xyz_soll/1 -> Demux/1
  Demux/1 -> Sum2/1
  Demux/2 -> Sum3/1

== system quad_model_control/Controller/sfun_controller/Constant_Subsystem ==
  In1 : Inport
  Constant : Constant  Value=0  OutDataTypeStr=single
  Out1 : Outport

== matlab function quad_model_control/kinematik/MATLAB Function ==
  data: om input; Phi_dot output; Phi input
function Phi_dot = eulerRates(om, Phi)
phi = Phi(1); the = Phi(2);
sph=sin(phi); cph=cos(phi); cth=cos(the); tth=tan(the);
W = [1, sph*tth, cph*tth;
     0, cph,    -sph;
     0, sph/cth, cph/cth];   % Singularität bei the = ±pi/2
Phi_dot = W * om;
end

== matlab function quad_model_control/dynamik_6DoF/MATLAB Function ==
  data: F_ext input; v_dot output; M_b input; v_b input; om input; Phi input; m input; g input; Ivec input; om_dot output
function [v_dot, om_dot] = eom_rhs(F_ext, M_b, v_b, om, Phi, m, g, Ivec)
% ... R weiterhin intern berechnen (für die Gravitation!) ...
phi=Phi(1); the=Phi(2); psi=Phi(3);
cph=cos(phi); sph=sin(phi); cth=cos(the); sth=sin(the); cps=cos(psi); sps=sin(psi);
R = [cth*cps, sph*sth*cps-cph*sps, cph*sth*cps+sph*sps;
     cth*sps, sph*sth*sps+cph*cps, cph*sth*sps-sph*cps;
    -sth,     sph*cth,             cph*cth];
F_grav_b = R.' * [0; 0; m*g];
v_dot  = (F_ext + F_grav_b)/m - cross(om, v_b);   % (4.1)
om_dot = (M_b - cross(om, Ivec.*om)) ./ Ivec;     % (4.2)
end

== matlab function quad_model_control/kinematik/MATLAB Function1 ==
  data: R output; Phi input
function R = buildR(Phi)
phi=Phi(1); the=Phi(2); psi=Phi(3);
cph=cos(phi); sph=sin(phi); cth=cos(the); sth=sin(the); cps=cos(psi); sps=sin(psi);
R = [cth*cps, sph*sth*cps-cph*sps, cph*sth*cps+sph*sps;
     cth*sps, sph*sth*sps+cph*cps, cph*sth*sps-sph*cps;
    -sth,     sph*cth,             cph*cth];
end
